simulink model "Separador_banda"  (R2017b)
settings: Solver=VariableStepAuto  StartTime=0.0  StopTime=30000  RelTol=1e-3
values from neighbouring files (symbols this model uses):
  hl = 2    [banda_separador.m]
  I1 = x(2)    [banda_separador.m]
  I3 = x(5)    [banda_separador.m]
  k1 = sym2poly(Ff_lo * Flo_xl)/a    [banda_separador.m]
  k2 = sym2poly(Ff_li)/a    [banda_separador.m]
  k3 = sym2poly(Ff_lo * Flo_p)/a    [banda_separador.m]
  k4 = sym2poly(Fg_li) /den    [banda_separador.m]
  k5 = sym2poly(Fg_gi)/den    [banda_separador.m]
  k6 = sym2poly(Fg_lo* Flo_xl) /den    [banda_separador.m]
  k7 = sym2poly((Fg_lo* Flo_hl)+(Fg_vl*Fvl_hl))/den    [banda_separador.m]
  k8 = sym2poly(Fg_go* Fgo_xg) /den    [banda_separador.m]
  k9 = sym2poly(Fg_go* Fgo_t) /den    [banda_separador.m]
  p = 8    [banda_separador.m]
  P1 = x(1)    [banda_separador.m]
  P2 = x(3)    [banda_separador.m]
  P3 = x(4)    [banda_separador.m]
  P4 = x(6)    [banda_separador.m]
  tau1 = 1/a    [banda_separador.m]
  tau2 = 1/a    [banda_separador.m]
  tau3 = tau1    [banda_separador.m]
  tau4 = 1 /den    [banda_separador.m]
  tau5 = tau4    [banda_separador.m]
  tau6 = tau4    [banda_separador.m]
  tau7 = tau4    [banda_separador.m]
  tau8 = tau4    [banda_separador.m]
  tau9 = tau4    [banda_separador.m]
libraries: simulink x4
settings Model: Creator=Rafael Azambuja  LastModifiedBy=Rafael Azambuja

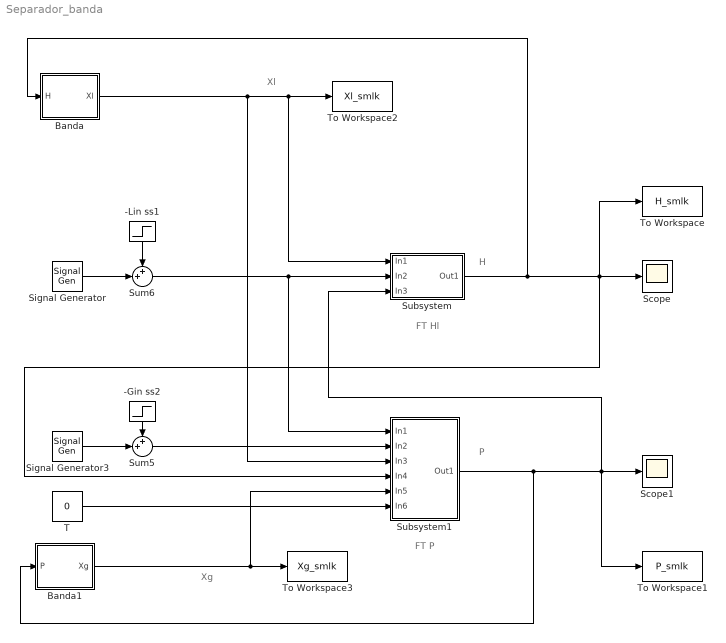
== system Separador_banda ==
  note: P
  note: Xg
  note: FT P
  note: H
  note: FT Hl
  note: Xl
  -Gin ss2 : Step  Time=0  After=0  SampleTime=0
  -Lin ss1 : Step  Time=0  After=0  SampleTime=0
  Banda : Subsystem
  Banda1 : Subsystem
  Scope : Scope
  Scope1 : Scope
  Signal Generator : SignalGenerator  Amplitude=0.05  Frequency=1/1320
  Signal Generator3 : SignalGenerator  Amplitude=0.0928  Frequency=1/1320
  Subsystem : Subsystem
  Subsystem1 : Subsystem
  Sum5 : Sum  Inputs=++|
  Sum6 : Sum  Inputs=++|
  T : Constant  Value=0
  To Workspace : ToWorkspace  VariableName=H_smlk  SaveFormat=Timeseries  SampleTime=1
  To Workspace1 : ToWorkspace  VariableName=P_smlk  SaveFormat=Timeseries  SampleTime=1
  To Workspace2 : ToWorkspace  VariableName=Xl_smlk  SaveFormat=Timeseries  SampleTime=1
  To Workspace3 : ToWorkspace  VariableName=Xg_smlk  SaveFormat=Timeseries  SampleTime=1
  wires:
  Sum6/1 -> Subsystem1/1(In1), Subsystem/2(In2)
  Banda/1(Xl) -> Subsystem1/3(In3), Subsystem/1(In1), To Workspace2/1
  Sum5/1 -> Subsystem1/2(In2)
  Signal Generator3/1 -> Sum5/2
  T/1 -> Subsystem1/6(In6)
  Signal Generator/1 -> Sum6/2
  -Lin ss1/1 -> Sum6/1
  Subsystem/1(Out1) -> Banda/1(H), To Workspace/1, Scope/1, Subsystem1/4(In4)
  -Gin ss2/1 -> Sum5/1
  Banda1/1(Xg) -> To Workspace3/1, Subsystem1/5(In5)
  Subsystem1/1(Out1) -> Banda1/1(P), To Workspace1/1, Scope1/1, Subsystem/3(In3)

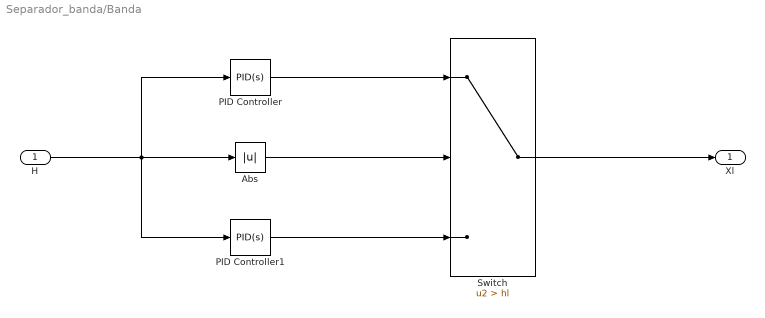
== system Separador_banda/Banda ==
  H : Inport
  Abs : Abs
  PID Controller : simulink/Continuous/PID Controller  Controller=PID  TimeDomain=Continuous-time  SampleTime=-1  IntegratorMethod=Forward Euler  FilterMethod=Forward Euler  Form=Parallel  UseFilter=on  ControllerParametersSource=internal  P=P1  I=I1  D=0  N=0  InitialConditionSource=internal  InitialConditionForIntegrator=0  InitialConditionForFilter=0  ExternalReset=none  LimitOutput=off  UpperSaturationLimit=inf  LowerSaturationLimit=-inf  LinearizeAsGain=on  AntiWindupMode=none  Kb=1  TrackingMode=off  Kt=1  PParamMin=[]  PParamMax=[]  IParamMin=[]  IParamMax=[]  DParamMin=[]  DParamMax=[]  NParamMin=[]  NParamMax=[]  KbParamMin=[]  KbParamMax=[]  KtParamMin=[]  KtParamMax=[]  POutMin=[]  POutMax=[]  IOutMin=[]  IOutMax=[]  DOutMin=[]  DOutMax=[]  NOutMin=[]  NOutMax=[]  KbOutMin=[]  KbOutMax=[]  KtOutMin=[]  KtOutMax=[]  IntegratorOutMin=[]  IntegratorOutMax=[]  FilterOutMin=[]  FilterOutMax=[]  SumOutMin=[]  SumOutMax=[]  SumI1OutMin=[]  SumI1OutMax=[]  SumI2OutMin=[]  SumI2OutMax=[]  SumI3OutMin=[]  SumI3OutMax=[]  SumDOutMin=[]  SumDOutMax=[]  SaturationOutMin=[]  SaturationOutMax=[]  IntegratorContinuousStateAttributes=''  IntegratorStateMustResolveToSignalObject=off  IntegratorRTWStateStorageClass=Auto  FilterContinuousStateAttributes=''  FilterStateMustResolveToSignalObject=off  FilterRTWStateStorageClass=Auto  DifferentiatorICPrevScaledInput=0  DifferentiatorOutMin=[]  DifferentiatorOutMax=[]  InitialConditionSetting=State (most efficient)  FilterDiffOutCoefMin=[]  FilterDiffOutCoefMax=[]  SumDenOutMin=[]  SumDenOutMax=[]  SumNumOutMin=[]  SumNumOutMax=[]  ReciprocalOutMin=[]  ReciprocalOutMax=[]  DivideOutMin=[]  DivideOutMax=[]  TunerSelectOption=Transfer Function Based (PID Tuner App)
  PID Controller1 : simulink/Continuous/PID Controller  Controller=PID  TimeDomain=Continuous-time  SampleTime=-1  IntegratorMethod=Forward Euler  FilterMethod=Forward Euler  Form=Parallel  UseFilter=on  ControllerParametersSource=internal  P=P2  I=0  D=0  N=0  InitialConditionSource=internal  InitialConditionForIntegrator=0  InitialConditionForFilter=0  ExternalReset=none  LimitOutput=off  UpperSaturationLimit=inf  LowerSaturationLimit=-inf  LinearizeAsGain=on  AntiWindupMode=none  Kb=1  TrackingMode=off  Kt=1  PParamMin=[]  PParamMax=[]  IParamMin=[]  IParamMax=[]  DParamMin=[]  DParamMax=[]  NParamMin=[]  NParamMax=[]  KbParamMin=[]  KbParamMax=[]  KtParamMin=[]  KtParamMax=[]  POutMin=[]  POutMax=[]  IOutMin=[]  IOutMax=[]  DOutMin=[]  DOutMax=[]  NOutMin=[]  NOutMax=[]  KbOutMin=[]  KbOutMax=[]  KtOutMin=[]  KtOutMax=[]  IntegratorOutMin=[]  IntegratorOutMax=[]  FilterOutMin=[]  FilterOutMax=[]  SumOutMin=[]  SumOutMax=[]  SumI1OutMin=[]  SumI1OutMax=[]  SumI2OutMin=[]  SumI2OutMax=[]  SumI3OutMin=[]  SumI3OutMax=[]  SumDOutMin=[]  SumDOutMax=[]  SaturationOutMin=[]  SaturationOutMax=[]  IntegratorContinuousStateAttributes=''  IntegratorStateMustResolveToSignalObject=off  IntegratorRTWStateStorageClass=Auto  FilterContinuousStateAttributes=''  FilterStateMustResolveToSignalObject=off  FilterRTWStateStorageClass=Auto  DifferentiatorICPrevScaledInput=0  DifferentiatorOutMin=[]  DifferentiatorOutMax=[]  InitialConditionSetting=State (most efficient)  FilterDiffOutCoefMin=[]  FilterDiffOutCoefMax=[]  SumDenOutMin=[]  SumDenOutMax=[]  SumNumOutMin=[]  SumNumOutMax=[]  ReciprocalOutMin=[]  ReciprocalOutMax=[]  DivideOutMin=[]  DivideOutMax=[]  TunerSelectOption=Transfer Function Based (PID Tuner App)
  Switch : Switch  Criteria=u2 > Threshold  Threshold=hl
  Xl : Outport
  wires:
  Abs/1 -> Switch/2
  H/1 -> PID Controller1/1, PID Controller/1, Abs/1
  PID Controller/1 -> Switch/1
  PID Controller1/1 -> Switch/3
  Switch/1 -> Xl/1

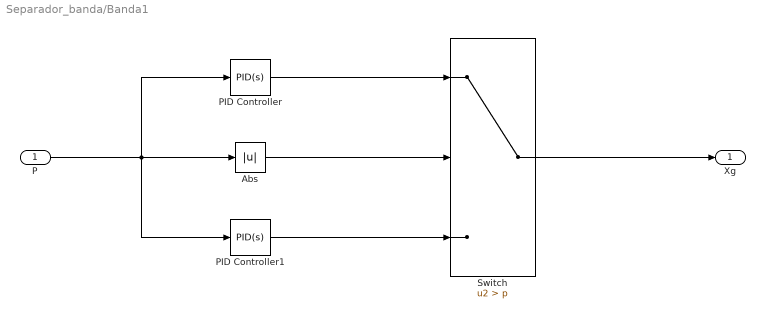
== system Separador_banda/Banda1 ==
  P : Inport
  Abs : Abs
  PID Controller : simulink/Continuous/PID Controller  Controller=PID  TimeDomain=Continuous-time  SampleTime=-1  IntegratorMethod=Forward Euler  FilterMethod=Forward Euler  Form=Parallel  UseFilter=on  ControllerParametersSource=internal  P=P3  I=I3  D=0  N=0  InitialConditionSource=internal  InitialConditionForIntegrator=0  InitialConditionForFilter=0  ExternalReset=none  LimitOutput=off  UpperSaturationLimit=inf  LowerSaturationLimit=-inf  LinearizeAsGain=on  AntiWindupMode=none  Kb=1  TrackingMode=off  Kt=1  PParamMin=[]  PParamMax=[]  IParamMin=[]  IParamMax=[]  DParamMin=[]  DParamMax=[]  NParamMin=[]  NParamMax=[]  KbParamMin=[]  KbParamMax=[]  KtParamMin=[]  KtParamMax=[]  POutMin=[]  POutMax=[]  IOutMin=[]  IOutMax=[]  DOutMin=[]  DOutMax=[]  NOutMin=[]  NOutMax=[]  KbOutMin=[]  KbOutMax=[]  KtOutMin=[]  KtOutMax=[]  IntegratorOutMin=[]  IntegratorOutMax=[]  FilterOutMin=[]  FilterOutMax=[]  SumOutMin=[]  SumOutMax=[]  SumI1OutMin=[]  SumI1OutMax=[]  SumI2OutMin=[]  SumI2OutMax=[]  SumI3OutMin=[]  SumI3OutMax=[]  SumDOutMin=[]  SumDOutMax=[]  SaturationOutMin=[]  SaturationOutMax=[]  IntegratorContinuousStateAttributes=''  IntegratorStateMustResolveToSignalObject=off  IntegratorRTWStateStorageClass=Auto  FilterContinuousStateAttributes=''  FilterStateMustResolveToSignalObject=off  FilterRTWStateStorageClass=Auto  DifferentiatorICPrevScaledInput=0  DifferentiatorOutMin=[]  DifferentiatorOutMax=[]  InitialConditionSetting=State (most efficient)  FilterDiffOutCoefMin=[]  FilterDiffOutCoefMax=[]  SumDenOutMin=[]  SumDenOutMax=[]  SumNumOutMin=[]  SumNumOutMax=[]  ReciprocalOutMin=[]  ReciprocalOutMax=[]  DivideOutMin=[]  DivideOutMax=[]  TunerSelectOption=Transfer Function Based (PID Tuner App)
  PID Controller1 : simulink/Continuous/PID Controller  Controller=PID  TimeDomain=Continuous-time  SampleTime=-1  IntegratorMethod=Forward Euler  FilterMethod=Forward Euler  Form=Parallel  UseFilter=on  ControllerParametersSource=internal  P=P4  I=0  D=0  N=0  InitialConditionSource=internal  InitialConditionForIntegrator=0  InitialConditionForFilter=0  ExternalReset=none  LimitOutput=off  UpperSaturationLimit=inf  LowerSaturationLimit=-inf  LinearizeAsGain=on  AntiWindupMode=none  Kb=1  TrackingMode=off  Kt=1  PParamMin=[]  PParamMax=[]  IParamMin=[]  IParamMax=[]  DParamMin=[]  DParamMax=[]  NParamMin=[]  NParamMax=[]  KbParamMin=[]  KbParamMax=[]  KtParamMin=[]  KtParamMax=[]  POutMin=[]  POutMax=[]  IOutMin=[]  IOutMax=[]  DOutMin=[]  DOutMax=[]  NOutMin=[]  NOutMax=[]  KbOutMin=[]  KbOutMax=[]  KtOutMin=[]  KtOutMax=[]  IntegratorOutMin=[]  IntegratorOutMax=[]  FilterOutMin=[]  FilterOutMax=[]  SumOutMin=[]  SumOutMax=[]  SumI1OutMin=[]  SumI1OutMax=[]  SumI2OutMin=[]  SumI2OutMax=[]  SumI3OutMin=[]  SumI3OutMax=[]  SumDOutMin=[]  SumDOutMax=[]  SaturationOutMin=[]  SaturationOutMax=[]  IntegratorContinuousStateAttributes=''  IntegratorStateMustResolveToSignalObject=off  IntegratorRTWStateStorageClass=Auto  FilterContinuousStateAttributes=''  FilterStateMustResolveToSignalObject=off  FilterRTWStateStorageClass=Auto  DifferentiatorICPrevScaledInput=0  DifferentiatorOutMin=[]  DifferentiatorOutMax=[]  InitialConditionSetting=State (most efficient)  FilterDiffOutCoefMin=[]  FilterDiffOutCoefMax=[]  SumDenOutMin=[]  SumDenOutMax=[]  SumNumOutMin=[]  SumNumOutMax=[]  ReciprocalOutMin=[]  ReciprocalOutMax=[]  DivideOutMin=[]  DivideOutMax=[]  TunerSelectOption=Transfer Function Based (PID Tuner App)
  Switch : Switch  Criteria=u2 > Threshold  Threshold=p
  Xg : Outport
  wires:
  Abs/1 -> Switch/2
  P/1 -> PID Controller1/1, PID Controller/1, Abs/1
  PID Controller/1 -> Switch/1
  PID Controller1/1 -> Switch/3
  Switch/1 -> Xg/1

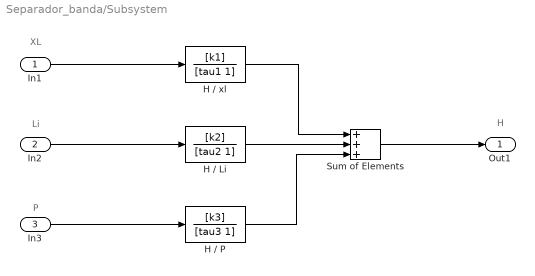
== system Separador_banda/Subsystem ==
  note: H
  note: P
  note: Li
  note: XL
  In1 : Inport
  In2 : Inport  Port=2
  In3 : Inport  Port=3
  H / Li : TransferFcn  Numerator=[k2]  Denominator=[tau2 1]
  H / P : TransferFcn  Numerator=[k3]  Denominator=[tau3 1]
  H / xl : TransferFcn  Numerator=[k1]  Denominator=[tau1 1]
  Sum of Elements : Sum  Inputs=+++
  Out1 : Outport
  wires:
  In1/1 -> H / xl/1
  In2/1 -> H / Li/1
  In3/1 -> H / P/1
  H / xl/1 -> Sum of Elements/1
  H / Li/1 -> Sum of Elements/2
  H / P/1 -> Sum of Elements/3
  Sum of Elements/1 -> Out1/1

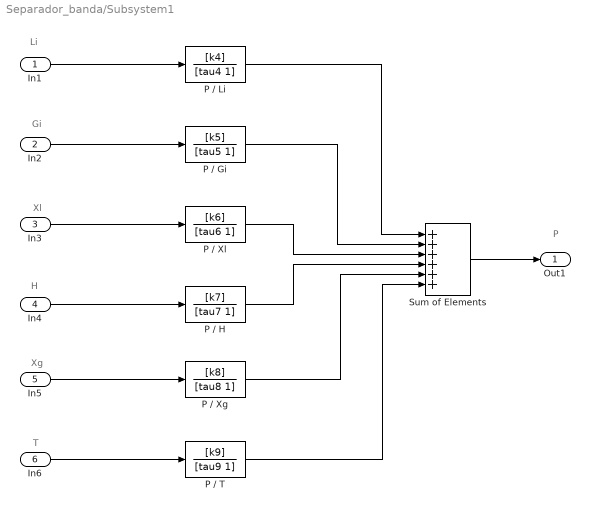
== system Separador_banda/Subsystem1 ==
  note: T
  note: Xg
  note: H
  note: P
  note: Xl
  note: Gi
  note: Li
  In1 : Inport
  In2 : Inport  Port=2
  In3 : Inport  Port=3
  In4 : Inport  Port=4
  In5 : Inport  Port=5
  In6 : Inport  Port=6
  P / Gi : TransferFcn  Numerator=[k5]  Denominator=[tau5 1]
  P / H : TransferFcn  Numerator=[k7]  Denominator=[tau7 1]
  P / Li : TransferFcn  Numerator=[k4]  Denominator=[tau4 1]
  P / T : TransferFcn  Numerator=[k9]  Denominator=[tau9 1]
  P / Xg : TransferFcn  Numerator=[k8]  Denominator=[tau8 1]
  P / Xl : TransferFcn  Numerator=[k6]  Denominator=[tau6 1]
  Sum of Elements : Sum  Inputs=++++++
  Out1 : Outport
  wires:
  In1/1 -> P / Li/1
  In2/1 -> P / Gi/1
  In3/1 -> P / Xl/1
  Sum of Elements/1 -> Out1/1
  In4/1 -> P / H/1
  In5/1 -> P / Xg/1
  In6/1 -> P / T/1
  P / T/1 -> Sum of Elements/6
  P / Xg/1 -> Sum of Elements/5
  P / H/1 -> Sum of Elements/4
  P / Xl/1 -> Sum of Elements/3
  P / Gi/1 -> Sum of Elements/2
  P / Li/1 -> Sum of Elements/1
